simulink model "milestone3"  (R2021a)
settings: Solver=FixedStepDiscrete  StartTime=0.0  StopTime=100  FixedStep=0.01  RelTol=1e-3
undefined symbols (not defined in the file): axleLength, DiscIntNeverNeededParam, InputPWM, lineLength, mapForSim, wheelR, WheelSpeed
libraries: mobileRoboticsTrainingLib x7, pid_lib x1
settings Model: EnablePacing=on  PacingRate=0.400000  Creator=Boitumelo  LastModifiedBy=Amandla Mvimbi

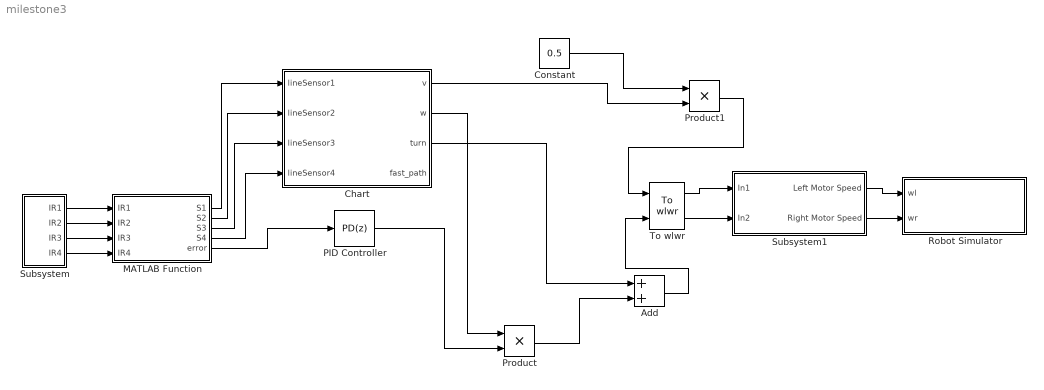
== system milestone3 ==
  Add : Sum
  Chart : Stateflow chart  TreatAsAtomicUnit=on
      settings: PortSchema="{\"entries\":[{\"content\":{\"sides\":[{\"content\":{\"connectorIds\":[\"In2\",\"In1\",\"In3\",\"In4\"]},\"type\":\"ConnectorPlacement.EquallySpacedRectSide\",\"uuid\":\"d58bfd7d-d9aa-44ac-a886-e1ac0f84a218\"},{\"content\":{\"connectorIds\":[\"Out2\",\"Out1\",\"Out3\",\"Out4\"],\"side\":\"RIGHT\"},\"type\":\"ConnectorPlacement.EquallySpacedRectSide\",\"uuid\":\"8746f1c2-b2f6-4eb2-9f38-8eacad1c9f3f\"},{\"content\":{\"connectorIds\":[],\"side\":\"TOP\"},\"type\":\"ConnectorPlacement.EquallySpacedRectSide\",\"uuid\":\"701b2a97-2393-4f89-9725-04fa9c7d6a07\"}]},\"type\":\"ConnectorPlacement.EquallySpacedConnector\",\"uuid\":\"55d5f9d3-4145-4892-80a0-0480acf37473\"}],\"packageUris\":[\"http://schema.mathworks.com/mf0/Connector/R2020b\"],\"version\":\"1.0\"}"
  Constant : Constant  Value=0.5
  MATLAB Function : MATLAB Function  TreatAsAtomicUnit=on
  PID Controller : pid_lib/PID Controller  Controller=PD  Form=Parallel  TimeDomain=Discrete-time  UseExternalTs=off  SampleTime=-1  IntegratorMethod=Forward Euler  FilterMethod=Forward Euler  ControllerParametersSource=internal  P=5  I=1  D=1e-5  UseFilter=on  N=100  TunerSelectOption=Transfer Function Based (PID Tuner App)  InitialConditionSource=internal  InitialConditionForIntegrator=0  InitialConditionForFilter=0  DifferentiatorICPrevScaledInput=0  ExternalReset=none  TrackingMode=off  Kt=1  LimitOutput=off  SatLimitsSource=internal  UpperSaturationLimit=inf  LowerSaturationLimit=-inf  LinearizeAsGain=on  AntiWindupMode=none  Kb=1  POutMin=[]  POutMax=[]  IOutMin=[]  IOutMax=[]  DOutMin=[]  DOutMax=[]  NOutMin=[]  NOutMax=[]  SumOutMin=[]  SumOutMax=[]  SaturationOutMin=[]  SaturationOutMax=[]  PParamMin=[]  PParamMax=[]  IParamMin=[]  IParamMax=[]  DParamMin=[]  DParamMax=[]  NParamMin=[]  NParamMax=[]  KbParamMin=[]  KbParamMax=[]  KtParamMin=[]  KtParamMax=[]  KbOutMin=[]  KbOutMax=[]  KtOutMin=[]  KtOutMax=[]  IntegratorOutMin=[]  IntegratorOutMax=[]  FilterOutMin=[]  FilterOutMax=[]  SumI1OutMin=[]  SumI1OutMax=[]  SumI2OutMin=[]  SumI2OutMax=[]  SumI3OutMin=[]  SumI3OutMax=[]  SumI4OutMin=[]  SumI4OutMax=[]  SumDOutMin=[]  SumDOutMax=[]  DifferentiatorOutMin=[]  DifferentiatorOutMax=[]  FilterDiffOutCoefMin=[]  FilterDiffOutCoefMax=[]  ReciprocalOutMin=[]  ReciprocalOutMax=[]  SumDenOutMin=[]  SumDenOutMax=[]  SumNumOutMin=[]  SumNumOutMax=[]  DivideOutMin=[]  DivideOutMax=[]  UdiffTsProdOutMin=[]  UdiffTsProdOutMax=[]  NTsProdOutMin=[]  NTsProdOutMax=[]  UintegralTsProdOutMin=[]  UintegralTsProdOutMax=[]  UngainTsProdOutMin=[]  UngainTsProdOutMax=[]  IntegratorContinuousStateAttributes=''  IntegratorStateMustResolveToSignalObject=off  IntegratorRTWStateStorageClass=Auto  FilterContinuousStateAttributes=''  FilterStateMustResolveToSignalObject=off  FilterRTWStateStorageClass=Auto  ParallelPVariant=InternalParameters  IdealPVariant=Disabled  IVariant=Disabled  DVariant=InternalParameters  IntegratorVariant=Disabled  SatVariant=Disabled  AWVariant=Disabled  PCopyVariant=Disabled  TRVariant=Disabled  FdbkBlocksVariant=Forward  IdealPFdbkVariant=Disabled  SatFdbkVariant=Disabled  DerivativeFilterVariant=ForwardEulerFilter  NVariant=InternalParameters  NCopyVariant=Disabled  FilterICVariant=InternalICsFilter  IntegratorICVariant=Disabled  ExternalResetVariant=Disabled  TRSumVariant=Passthrough  SumFdbkVariant=Disabled  SumVariant=Sum_PD  TsampFilterVariant=InternalTs  TsampNgainVariant=Passthrough  TsampIntegralVariant=Disabled_SignalSpec  ExternalSaturationOutDataTypeStr=Inherit: Same as second input
  Product : Product
  Product1 : Product
  Robot Simulator : Subsystem  Priority=99  AncestorBlock=mobileRoboticsTrainingLib/Robot Simulator  mask(Robot Simulator){mapVar=mapForSim, startX=0.13698, startY=0.092707, startTheta=0, axleLength=axleLength, wheelR=wheelR}
      mask prompts: mapVar "Map Variable"; startX "Start X (m)"; startY "Start Y (m)"; startTheta "Theta (deg)"; axleLength "Axle Length (m)"; wheelR "Wheel Radius (m)"
      mask help: Configure robot simulator to use custom simulation maps and simulate closed-loop mobile robotics systems along with appropriate sensor simulation blocks.
      mask init:
      | set_param(bdroot,'SolverType','Fixed-Step');
      | set_param(bdroot,'Solver','FixedStepDiscrete');
      | 
      | if (exist('Ts'))
      |     set_param(bdroot,'FixedStep','Ts');
      | else
      |     set_param(bdroot,'FixedStep','0.01');
      | end
      | 
      | h = findobj('Name','Robot Simulator');
      | if ~isempty(h)
      |     close (h);
      | end
      | setupRobotSim();
      mask Help: web('Robot Simulator.htm')
      mask DialogControl mapCont Prompt: Map Setup
      mask DialogControl initPosCont Prompt: Initial Position
      mask DialogControl setPos Prompt: Set position interactively
      mask DialogControl setPos Callback:
      | %% Set starting point
      | setStartingPoint();
      mask DialogControl initOrientation Prompt: Initial Orientation
      mask DialogControl robotCharCont Prompt: Robot Characteristics
      mask Display: disp('Robot Simulator')
  Subsystem : Subsystem
  Subsystem1 : Subsystem
  To wlwr : mobileRoboticsTrainingLib/To wlwr  axleLength=0.1  wheelR=0.05
  wires:
  MATLAB Function/4(S4) -> Chart/4(lineSensor4)
  MATLAB Function/3(S3) -> Chart/3(lineSensor3)
  MATLAB Function/2(S2) -> Chart/1(lineSensor2)
  MATLAB Function/1(S1) -> Chart/2(lineSensor1)
  Product1/1 -> To wlwr/1
  Constant/1 -> Product1/1
  Add/1 -> To wlwr/2
  Chart/2(v) -> Product1/2
  Chart/1(w) -> Product/1
  Chart/3(turn) -> Add/1
  Product/1 -> Add/2
  PID Controller/1 -> Product/2
  MATLAB Function/5(error) -> PID Controller/1
  Subsystem/1(IR1) -> MATLAB Function/1(IR1)
  Subsystem/2(IR2) -> MATLAB Function/2(IR2)
  Subsystem/3(IR3) -> MATLAB Function/3(IR3)
  Subsystem/4(IR4) -> MATLAB Function/4(IR4)
  To wlwr/1 -> Subsystem1/1(In1)
  To wlwr/2 -> Subsystem1/2(In2)
  Subsystem1/1(Left Motor Speed) -> Robot Simulator/1(wl)
  Subsystem1/2(Right Motor Speed) -> Robot Simulator/2(wr)

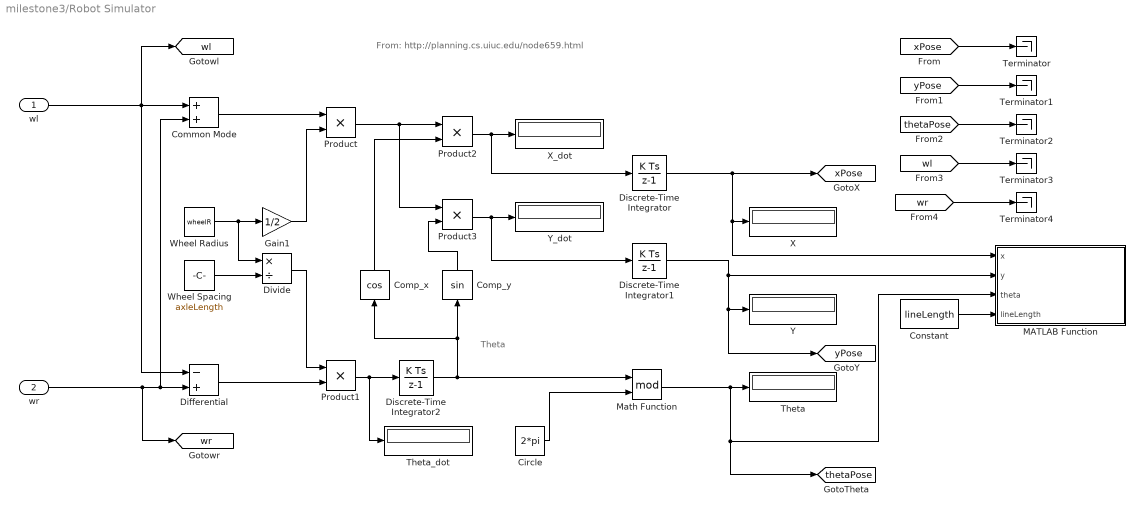
== system milestone3/Robot Simulator ==
  note: Theta
  note: From: http://planning.cs.uiuc.edu/node659.html
  wl : Inport
  wr : Inport  Port=2
  Circle : Constant  Value=2*pi
  Common Mode : Sum
  Comp_x : Trigonometry  Operator=cos
  Comp_y : Trigonometry
  Constant : Constant  Value=lineLength
  Differential : Sum  Inputs=-+
  Discrete-Time Integrator : DiscreteIntegrator  InitialCondition=startX  SampleTime=-1  ICPrevOutput=DiscIntNeverNeededParam  ICPrevScaledInput=DiscIntNeverNeededParam
  Discrete-Time Integrator1 : DiscreteIntegrator  InitialCondition=startY  SampleTime=-1  ICPrevOutput=DiscIntNeverNeededParam  ICPrevScaledInput=DiscIntNeverNeededParam
  Discrete-Time Integrator2 : DiscreteIntegrator  InitialCondition=startTheta*(pi/180)  SampleTime=-1  ICPrevOutput=DiscIntNeverNeededParam  ICPrevScaledInput=DiscIntNeverNeededParam
  Divide : Product  Inputs=*/
  Gain1 : Gain  Gain=1/2
  MATLAB Function : MATLAB Function  TreatAsAtomicUnit=on
  Math Function : Math  Operator=mod  SignedPower=on  SaturateOnIntegerOverflow=on
  Product{,1..3} (4 alike) : Product  RndMeth=Zero
  Terminator{,1..4} (5 alike) : Terminator
  Theta : Display
  Theta_dot : Display
  Wheel Radius : Constant  Value=wheelR
  Wheel Spacing : Constant  Value=axleLength
  X : Display
  X_dot : Display
  Y : Display
  Y_dot : Display
  tag scope: thetaPose=global, wl=global, wr=global, xPose=global, yPose=global
  wires:
  [wr] -> Terminator4/1
  [wl] -> Terminator3/1
  Math Function/1 -> [thetaPose], MATLAB Function/3(theta), Theta/1
  Differential/1 -> Product1/2
  Comp_y/1 -> Product3/2
  Discrete-Time Integrator/1 -> [xPose], MATLAB Function/1(x), X/1
  Product3/1 -> Discrete-Time Integrator1/1, Y_dot/1
  Discrete-Time Integrator1/1 -> Y/1, [yPose], MATLAB Function/2(y)
  Divide/1 -> Product1/1
  wr/1 -> [wr], Common Mode/2, Differential/2
  Discrete-Time Integrator2/1 -> Math Function/1, Comp_x/1, Comp_y/1
  wl/1 -> [wl], Common Mode/1, Differential/1
  Comp_x/1 -> Product2/2
  Product1/1 -> Discrete-Time Integrator2/1, Theta_dot/1
  Wheel Radius/1 -> Divide/1, Gain1/1
  Wheel Spacing/1 -> Divide/2
  Product2/1 -> Discrete-Time Integrator/1, X_dot/1
  Gain1/1 -> Product/2
  Common Mode/1 -> Product/1
  Product/1 -> Product3/1, Product2/1
  Circle/1 -> Math Function/2
  Constant/1 -> MATLAB Function/4(lineLength)
  [xPose] -> Terminator/1
  [yPose] -> Terminator1/1
  [thetaPose] -> Terminator2/1

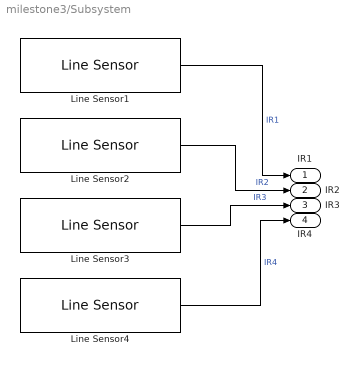
== system milestone3/Subsystem ==
  Line Sensor1 : mobileRoboticsTrainingLib/Line Sensor  mapVariable=mapForSim  envVal=2850  lineVal=2950  sensOff=[0.0643 0.0354]
      settings: SourceProductName=Mobile Robotics Training Library
  Line Sensor2 : mobileRoboticsTrainingLib/Line Sensor  mapVariable=mapForSim  envVal=2850  lineVal=2950  sensOff=[0.0675 0.005]
      settings: SourceProductName=Mobile Robotics Training Library
  Line Sensor3 : mobileRoboticsTrainingLib/Line Sensor  mapVariable=mapForSim  envVal=2850  lineVal=2950  sensOff=[0.0675 -0.005]
      settings: SourceProductName=Mobile Robotics Training Library
  Line Sensor4 : mobileRoboticsTrainingLib/Line Sensor  mapVariable=mapForSim  envVal=2850  lineVal=2950  sensOff=[0.0643 -0.0354]
      settings: SourceProductName=Mobile Robotics Training Library
  IR1 : Outport
  IR2 : Outport  Port=2
  IR3 : Outport  Port=3
  IR4 : Outport  Port=4
  wires:
  Line Sensor1/1 -> IR1/1  "IR1"
  Line Sensor2/1 -> IR2/1  "IR2"
  Line Sensor4/1 -> IR4/1  "IR4"
  Line Sensor3/1 -> IR3/1  "IR3"

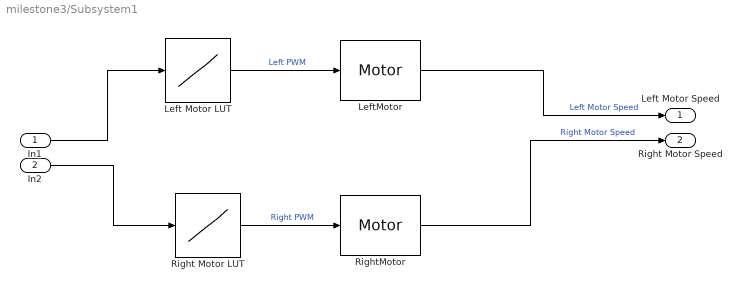
== system milestone3/Subsystem1 ==
  In1 : Inport
  In2 : Inport  Port=2
  Left Motor LUT : Lookup_n-D  NumberOfTableDimensions=1  BreakpointsForDimension1=WheelSpeed  Table=InputPWM  InterpMethod=Nearest  ExtrapMethod=Clip  InternalRulePriority=Speed  RndMeth=Simplest  InputSameDT=on
  LeftMotor : mobileRoboticsTrainingLib/Motor  motorPlant=wheelMotorModel  sensorType=Speed
      settings: SourceProductName=Mobile Robotics Training Library
  Right Motor LUT : Lookup_n-D  NumberOfTableDimensions=1  BreakpointsForDimension1=WheelSpeed  Table=InputPWM  InterpMethod=Nearest  ExtrapMethod=Clip  InternalRulePriority=Speed  RndMeth=Simplest  InputSameDT=on
  RightMotor : mobileRoboticsTrainingLib/Motor  motorPlant=wheelMotorModel  sensorType=Speed
      settings: SourceProductName=Mobile Robotics Training Library
  Left Motor Speed : Outport
  Right Motor Speed : Outport  Port=2
  wires:
  LeftMotor/1 -> Left Motor Speed/1  "Left Motor Speed"
  In1/1 -> Left Motor LUT/1
  RightMotor/1 -> Right Motor Speed/1  "Right Motor Speed"
  Left Motor LUT/1 -> LeftMotor/1  "Left PWM"
  In2/1 -> Right Motor LUT/1
  Right Motor LUT/1 -> RightMotor/1  "Right PWM"

== matlab function milestone3/Robot Simulator/MATLAB Function ==
  data: x input; y input; theta input; lineLength input
function plotRobot(x,y,theta,lineLength)
% Get plot details
coder.extrinsic('evalin','plot')
ph1 = evalin('base','PlotHandle1');
ph2 = evalin('base','PlotHandle2');

% Find length orientation line
xp = [x x+lineLength*cos(theta)];
yp = [y y+lineLength*sin(theta)];

% Plot robot
set(ph1,'xdata',xp,'ydata',yp);
set(ph2,'xdata',x,'ydata',y);
drawnow('limitrate')

== matlab function milestone3/MATLAB Function ==
  data: S1 output; S2 output; S3 output; S4 output; IR1 input; error output; IR2 input; IR3 input; IR4 input
function [S1, S2, S3, S4, error]= fcn(IR1, IR2, IR3, IR4)
% Sets the number of sensors on the line to 0
numberof0 = 0;
% Creates a persistent variable line
persistent line;
if isempty(line)
    line = "Line";
end
% Sets S1 to 0 if it is on the line and 1 if it is off
if IR1 >= 2900
    S1 = 0;
else
    S1 = 1;
end
% Sets S2 to 0 if it is on the line and 1 if it is off
if IR2 >= 2900
    S2 = 0;
    % Increments the count of number of sensors on the line
    numberof0 = numberof0 + 1;
else
    S2 = 1;
end
% Sets S3 to 0 if it is on the line and 1 if it is off
if IR3 >= 2900
    S3 = 0;
    % Increments the count of number of sensors on the line
    numberof0 = numberof0 + 1;
else
    S3 = 1;
end
% Sets S4 to 0 if it is on the line and 1 if it is off
if IR4 >= 2900
    S4 = 0;
else
    S4 = 1;
end
if numberof0 == 0
    CurrentDeveation = 0;
else
    CurrentDeveation = ((S2*2)+(S3*-2))/numberof0;  
end
error = 0 - CurrentDeveation;

== stateflow chart milestone3/Chart ==
  state Start
    entry:
    v=1;
    w=1;
    turn=0;
    length1=0;
    path = zeros(1,50);
    fast_path = zeros(1,50)
  state RightT
    entry:
    v=0;
    w=1;
    turn=0;
    path(length1)=1;
  state Junction_Detect
    entry:
    v=1;
    length1=length1+1;
  state Forward
    entry:
    v=1;
  state Right
    entry:
    v=0;
  state Right_Detect
    entry:
    v=0;
    w=0;
    turn=-1;
  state Left
    entry:
    v=0;
  state Straight
    entry:
    v=1;
  state Cross
  state Backward
    entry:
    v=1;
    w=1;
    turn=0;
    path(length1)=2;
  state Check
    entry:
    v=-0.5;
  state Check2
  state RightTurn
    entry:
    v=0;
    w=0;
    turn=-1;
  state Continue
    entry:
    v=1;
    w=1;
    turn=0;
    path(length1)=3;
  state Straight_Detect
    entry:
    v=0;
  state Left_Detect
    entry:
    v=0;
    w=0;
    turn=1;
  state Stop
    entry:
    v=0;
    w=0;
    turn=0;
    %fast_path = short_path(path,length1);
  state LeftT
    entry:
    v=0;
    w=1;
    turn=0;
    path(length1)=1;
  state LeftTurn
    entry:
    v=0;
    w=0;
    turn=1;
  state DeadEnd
    entry:
    v=0;
    w=0;
    turn=3;
  state TurnAround
    entry:
    v=0;
    w=0;
    turn=3;
  (default) -> Start
  Start -> Forward
  Continue -> Forward
  RightT -> Forward
  RightTurn -> RightT : [lineSensor2==0&&lineSensor3==0]
  Junction_Detect -> Right [order 1] : [lineSensor4 ==0]
  Forward -> Junction_Detect : [lineSensor1 == 0 || lineSensor2 == 1&& lineSensor3 == 1|| lineSensor4 == 0 ]
  Backward -> Forward
  Right -> Right_Detect [order 1] : [lineSensor4 ==0 && lineSensor2 ==1&& lineSensor3==1]
  LeftT -> Forward
  Junction_Detect -> Left [order 3] : [lineSensor1==0]
  Junction_Detect -> Straight [order 2] : after(0.1,sec)[lineSensor2==1&&lineSensor3==1]
  Right -> Continue [order 2] : after(0.3,sec)
  Right_Detect -> RightTurn : after(0.3,sec)
  Left -> Cross [order 2] : [lineSensor1==0&&lineSensor2==0&&lineSensor3==0&&lineSensor4==0]
  Left -> Check [order 1] : [lineSensor1==0&&lineSensor2==1&&lineSensor3==1]
  Cross -> Check2 : after(0.1,sec)
  Left -> Left_Detect [order 3]
  Straight -> Straight_Detect : after(0.2,sec)
  Straight_Detect -> Continue [order 2]
  Check -> Left_Detect : after(0.2,sec)
  Check2 -> Left_Detect [order 2]
  Check2 -> Stop [order 1] : [lineSensor1 == 0 && lineSensor2 == 0&& lineSensor3 == 0 && lineSensor4 == 0]
  TurnAround -> Backward : [lineSensor2==0&&lineSensor3==0]
  Straight_Detect -> DeadEnd [order 1] : [lineSensor1 == 1 && lineSensor2 == 1&& lineSensor3 == 1 && lineSensor4 == 1]
  Left_Detect -> LeftTurn : after(0.3,sec)
  LeftTurn -> LeftT : [lineSensor2==0&&lineSensor3==0]
  DeadEnd -> TurnAround : after(0.2,sec)
  data: num function_input; length function_input; short function_output; w output; lineSensor2 input; lineSensor1 input; lineSensor3 input; lineSensor4 input; v output; turn output; path_length local; path local; s_path local; length1 local; fast_path output
  function short = shortestpath(num, length):
    | function short = shortestpath(num, length)
    | patharray = zeros(1,length);
    | u = 1;
    | while u <= (length)
    |     x1 = num(u);
    |     x2 = num(u+1);
    |     x3 = num(u+2);
    |     if x1 == 1 && x2 == 2 && x3 == 4
    |         patharray(u) = 2;
    |         u = u+3;
    |     elseif x1 == 1 && x2 == 2 && x3 == 3
    |         patharray(u) = 4;
    |         u = u+3;
    |     elseif x1 == 4 && x2 == 2 && x3 == 1
    |         patharray(u) = 2;
    |         u = u+3;
    |     elseif x1 == 3 && x2 == 2 && x3 == 1
    |         patharray(u) = 4;
    |         u = u+3;
    |     elseif x1 == 3 && x2 == 2 && x3 == 3
    |         patharray(u) = 2;
    |         u = u+3;
    |     elseif x1 == 1 && x2 == 2 && x3 == 1
    |         patharray(u) = 3;
    |         u = u+3;
    |     else
    |         patharray(u) = x1;
    |         u = u+1;
    |     end
    |     if u == (length)
    |         for i = 1:length
    |             if patharray(u) == 2
    |                 u = 1;
    |                 num = patharray;
    |             end    
    |         end    
    |     end
    | end
    | disp(patharray);
    | short = patharray;
